simulink model "ParametricRobotWithGripperPayloads"  (R2023a)
settings: Solver=VariableStepAuto  StartTime=0.0  StopTime=10  RelTol=1e-3  AbsTol=1e-3  EnableMultiTasking=on
PostLoadFcn:
  | ParametricRobotParameters
  | ParametricGripperPayloadsParameters
undefined symbols (not defined in the file): X, Y, Z
libraries: sm_lib x3, fl_lib x2, nesl_utility x1
settings Model: Creator=abirdas  LastModifiedBy=abirdas
settings SolverCC: AutoScaleAbsTol=off  AlgebraicLoopSolver=TrustRegion  MaxZcPerStep=1
settings DataIOCC: LimitDataPoints=on  MaxDataPoints=10000
settings OptimizationCC: ReuseModelBlockBuffer=off  LifeSpan=inf
settings DebuggingCC: UnconnectedInputMsg=warning  UnconnectedOutputMsg=warning  UnconnectedLineMsg=warning  AllowSymbolicDim=off  SubsystemReferenceDiagnosticForUnitTest=warning  SFUnexpectedBacktrackingDiag=warning  SFNoUnconditionalDefaultTransitionDiag=warning  SFExecutionAtInitializationDiag=none  ArithmeticOperatorsInVariantConditions=warning
settings ModelReferenceCC: EnableRefExpFcnMdlSchedulingChecks=on
settings SFSimCC: SimUseLocalCustomCode=off  CustomCodeUndefinedFunction=UseInterfaceOnly
settings RTWCC: RTWUseLocalCustomCode=off  DLArmComputeVersion=19.05
settings CodeAppCC: StateflowObjectComments=on
settings GRTTargetCC: TargetLangStandard=C89/C90 (ANSI)
settings ConfigComp: CovMetricSettings=dw  CovSaveCumulativeToWorkspaceVar=on  CovSaveSingleToWorkspaceVar=on  CovExternalEMLEnable=off  CovSFcnEnable=off
settings SimscapeCC: SimscapeLogType=all  SimscapeLogSimulationStatistics=on  SimscapeLogDataHistory=10000

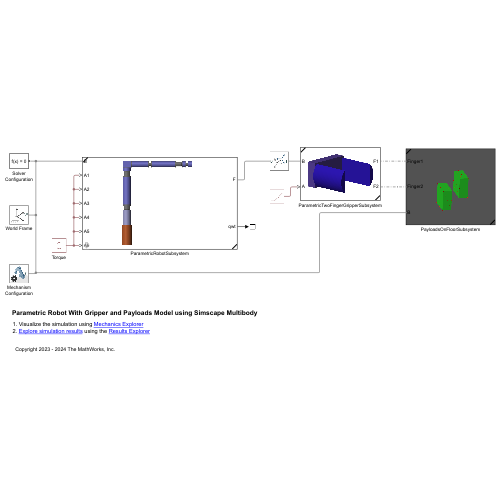
[thumbnail: Simulink's stored preview of the top-level diagram]
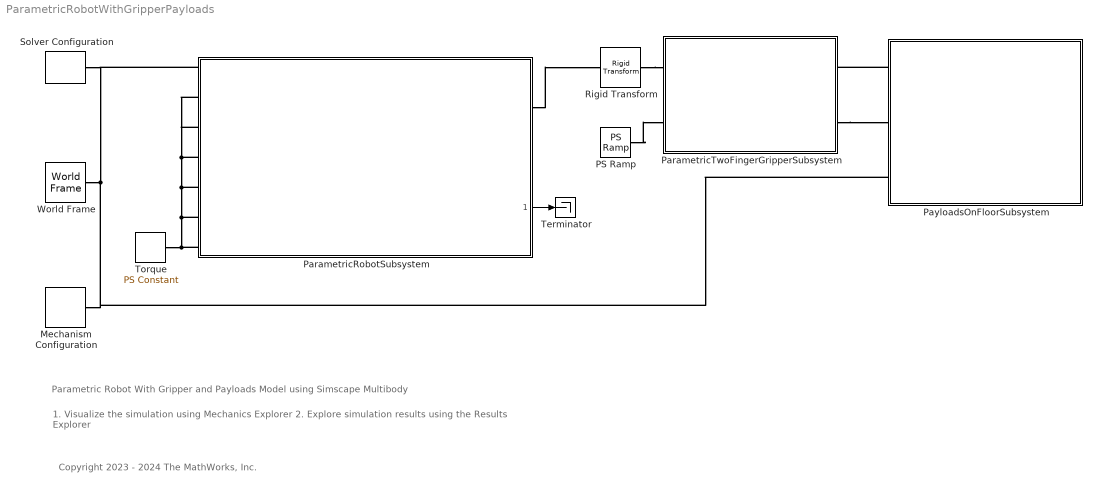
== system ParametricRobotWithGripperPayloads ==
  note: 1. Visualize the simulation using Mechanics Explorer
      | 2. Explore simulation results using the Results Explorer
  note: Parametric Robot With Gripper and Payloads Model using Simscape Multibody
  note: Copyright 2023 - 2024 The MathWorks, Inc.
  Mechanism Configuration : sm_lib/Utilities/Mechanism Configuration  UniformGravity=Constant  GravityVector=[0 0 -9.80665]  GravityVectorUnits=m/s^2  LinearizationDelta=0.001  JointModeTransitionNonlinearIterations=2
  PS Ramp : fl_lib/Physical Signals/Sources/PS Ramp  slope=0 N/s  start_time=0 s  initial_output=0 N
  ParametricRobotSubsystem : Subsystem  ReferencedSubsystem=ParametricRobotSubsystem  workflow=ones(1,6)
      settings: PortSchema="{\"entries\":[{\"content\":{\"sides\":[{\"content\":{\"connectorIds\":[\"LConn1\",\"LConn2\",\"LConn3\",\"LConn4\",\"LConn5\",\"LConn6\",\"LConn7\"]},\"type\":\"ConnectorPlacement.EquallySpacedRectSide\",\"uuid\":\"8e2b354c-8065-4b01-9993-90a522985fbc\"},{\"content\":{\"connectorIds\":[\"RConn1\",\"Out1\"],\"side\":\"RIGHT\"},\"type\":\"ConnectorPlacement.EquallySpacedRectSide\",\"uuid\":\"765c264f-d3d7-49d4-9ad7-cce0ed935f01\"},{\"content\":{\"side\":\"TOP\"},\"type\":\"ConnectorPlacement.EquallySpacedRectSide\",\"uuid\":\"138574ac-41af-40f6-ad96-19f9b89fa4a6\"}]},\"type\":\"ConnectorPlacement.EquallySpacedConnector\",\"uuid\":\"621780a5-4310-4379-a8cb-63d6a09a97de\"}],\"packageUris\":[\"http://schema.mathworks.com/mf0/Connector/R2020b\"],\"version\":\"1.0\"}"
  ParametricTwoFingerGripperSubsystem : Subsystem  ReferencedSubsystem=ParametricTwoFingerGripperSubsystem
  PayloadsOnFloorSubsystem : Subsystem  ReferencedSubsystem=PayloadsOnFloorSubsystem
  Rigid Transform : sm_lib/Frames and Transforms/Rigid Transform  TranslationMethod=None  TranslationStandardOffset=0  TranslationStandardOffsetUnits=m  TranslationStandardAxis=+Z  TranslationCartesianOffset=[0 0 0]  TranslationCartesianOffsetUnits=m  TranslationROffset=0  TranslationROffsetUnits=m  TranslationZOffset=0  TranslationZOffsetUnits=m  TranslationThetaOffset=0  TranslationThetaOffsetUnits=deg  RotationMethod=RotationSequence  RotationAngleUnits=deg  RotationStandardAxis=+Y  RotationAngle=90  RotationArbitraryAxis=[0 0 1]  FollAlignAxisA=+X  BaseAlignAxisA=+Y  FollAlignAxisB=+Y  BaseAlignAxisB=+Z  RotationSequenceAxes=BaseAxes  RotationSequence=XYZ  RotationSequenceAngles=[0 90 180]  RotationSequenceAnglesUnits=deg  RotationMatrix=[1 0 0; 0 1 0; 0 0 1]  Quaternion=[1 0 0 0]
  Solver Configuration : nesl_utility/Solver Configuration  PhysicalDomain=network_engine_domain  SubClassName=solver  LeftPortType=input  RightPortType=generic  Tones=[]  Harmonics=[]  SimulateNoise=off  Profile=off  UseLocalSampling=off  EnableSwitchedLinearOptims=on  FrequencyDomain=off  UseCCode=off  RelTol=0.001  AbsTol=1e-06  MinStep=1e-09  ToWorkspace=off  RevertToSquareIcSolve=off  NumHomotopyIterations=100  PhasorMode=off  PhasorModeNumHarmonics=1  ConsistencySolver=NEWTON_XTOL_AFTER_FTOL  IndexReductionMethod=DerivativeReplacement  DoDC=off  ResidualTolerance=1e-09  ConsistencyTolSource=GLOBAL  ConsistencyAbsTol=0.001  ConsistencyRelTol=0.001  ConsistencyTolFactor=0.001  UseLocalSolver=off  LocalSolverChoice=NE_BACKWARD_EULER_ADVANCER  ResolveIndetEquations=on  FunctionEvalNumThread=1  LocalSolverSampleTime=0.001  DoFixedCost=off  MaxNonlinIter=3  MaxModeIter=2  ComputeImpulses=off  ImpulseIterations=2  LinearAlgebra=Sparse  LinearAlgebraNumThread=0  EquationFormulation=NE_TIME_EF  DelaysMemoryBudget=1024  AutomaticFiltering=on  FilteringTimeConstant=0.001  PartitionStorageMethod=AS_NEEDED  PartitionMemoryBudget=1024  PartitionMethod=FAST
  Terminator : Terminator
  Torque : fl_lib/Physical Signals/Sources/PS Constant  constant=0 N*m
  World Frame : sm_lib/Frames and Transforms/World Frame
  wires:
  ParametricRobotSubsystem/1 -> Terminator/1
  connections:
  World Frame/RConn1 -- Solver Configuration/RConn1 -- ParametricRobotSubsystem/LConn1 -- PayloadsOnFloorSubsystem/LConn3 -- Mechanism Configuration/RConn1
  PayloadsOnFloorSubsystem/LConn1 -- ParametricTwoFingerGripperSubsystem/RConn1
  ParametricTwoFingerGripperSubsystem/RConn2 -- PayloadsOnFloorSubsystem/LConn2
  PS Ramp/RConn1 -- ParametricTwoFingerGripperSubsystem/LConn2
  ParametricRobotSubsystem/RConn1 -- Rigid Transform/LConn1
  Rigid Transform/RConn1 -- ParametricTwoFingerGripperSubsystem/LConn1
  Torque/RConn1 -- ParametricRobotSubsystem/LConn7 -- ParametricRobotSubsystem/LConn6 -- ParametricRobotSubsystem/LConn5 -- ParametricRobotSubsystem/LConn4 -- ParametricRobotSubsystem/LConn3 -- ParametricRobotSubsystem/LConn2
